simulink model "BLDC_Impedance_Controller"  (R2016a)
settings: Solver=VariableStepAuto  StartTime=0.0  StopTime=20  RelTol=1e-3
model workspace (MATLAB code in the model file):
  | J=0.000027; % Inertia kg/m^2
  | R=9.02; % Resistance Ohms
  | b=0.07; % Viscus damping NM/(rads/s)
  | Kt=0.63; % Torque Constant Nm/A
  | Ke=0.39; % Voltage constant V/(Rads/s)
  | L=0.0187; % Inductance H
  | m=0.1; % mass KG
  | G1= 0.1 % Saturation gain for friction model
  | g=9.81 % gravity m/sec^2
  | l=0.15 % length of arm in metres
libraries: simulink x2
settings Model: Creator=Lara  LastModifiedBy=mmdclm

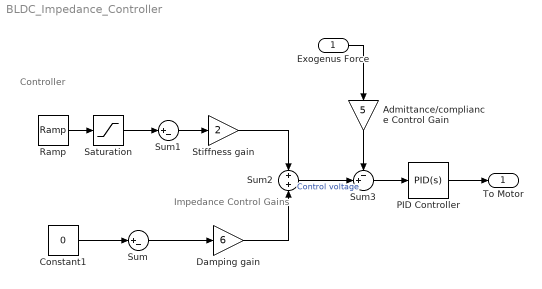
== system BLDC_Impedance_Controller ==
  note: Impedance Control
      | Gains
  note: Controller
  Exogenus Force : Inport
  Admittance/compliance Control Gain : Gain  Gain=5
  Constant1 : Constant  Value=0
  Damping gain : Gain  Gain=6
  PID Controller : simulink/Continuous/PID Controller  Controller=PID  TimeDomain=Continuous-time  SampleTime=-1  IntegratorMethod=Forward Euler  FilterMethod=Forward Euler  Form=Parallel  UseFilter=on  ControllerParametersSource=internal  P=0  I=0.731381886063385  D=0  N=100  InitialConditionSource=internal  InitialConditionForIntegrator=0  InitialConditionForFilter=0  ExternalReset=none  LimitOutput=off  UpperSaturationLimit=inf  LowerSaturationLimit=-inf  LinearizeAsGain=on  AntiWindupMode=none  Kb=1  TrackingMode=off  Kt=1  PParamMin=[]  PParamMax=[]  IParamMin=[]  IParamMax=[]  DParamMin=[]  DParamMax=[]  NParamMin=[]  NParamMax=[]  KbParamMin=[]  KbParamMax=[]  KtParamMin=[]  KtParamMax=[]  POutMin=[]  POutMax=[]  IOutMin=[]  IOutMax=[]  DOutMin=[]  DOutMax=[]  NOutMin=[]  NOutMax=[]  KbOutMin=[]  KbOutMax=[]  KtOutMin=[]  KtOutMax=[]  IntegratorOutMin=[]  IntegratorOutMax=[]  FilterOutMin=[]  FilterOutMax=[]  SumOutMin=[]  SumOutMax=[]  SumI1OutMin=[]  SumI1OutMax=[]  SumI2OutMin=[]  SumI2OutMax=[]  SumI3OutMin=[]  SumI3OutMax=[]  SumDOutMin=[]  SumDOutMax=[]  SaturationOutMin=[]  SaturationOutMax=[]  IntegratorContinuousStateAttributes=''  IntegratorStateMustResolveToSignalObject=off  IntegratorRTWStateStorageClass=Auto  FilterContinuousStateAttributes=''  FilterStateMustResolveToSignalObject=off  FilterRTWStateStorageClass=Auto  DifferentiatorICPrevScaledInput=0  DifferentiatorOutMin=[]  DifferentiatorOutMax=[]
  Ramp : simulink/Sources/Ramp  slope=10  start=0  X0=0
  Saturation : Saturate  UpperLimit=3.142
  Stiffness gain : Gain  Gain=2
  Sum : Sum  Inputs=|+-
  Sum1 : Sum  Inputs=|+-
  Sum2 : Sum  Inputs=+|+
  Sum3 : Sum  Inputs=-+|
  "To Motor " : Outport
  wires:
  Constant1/1 -> Sum/1
  Sum/1 -> Damping gain/1
  Sum1/1 -> Stiffness gain/1
  Stiffness gain/1 -> Sum2/1
  Damping gain/1 -> Sum2/2
  Sum2/1 -> Sum3/2  "Control voltage"
  Sum3/1 -> PID Controller/1
  Ramp/1 -> Saturation/1
  Saturation/1 -> Sum1/1
  Admittance/compliance Control Gain/1 -> Sum3/1
  Exogenus Force/1 -> Admittance/compliance Control Gain/1
  PID Controller/1 -> "To Motor "/1
